simulink model "gabelstapler_Simulink_25a"  (R2025a)
settings: Solver=VariableStepAuto  StartTime=0.0  StopTime=100  RelTol=1e-3
undefined symbols (not defined in the file): d, d_gtr, i_Getriebe, k, K_D, k_e, k_I, k_Motor, k_P, L_Motor, m_fz, m_g, m_gabel, R_Motor, r_R, theta_red, Wirkungsgad_Getriebe
settings Model: Creator=Manuel  LastModifiedBy=gerke

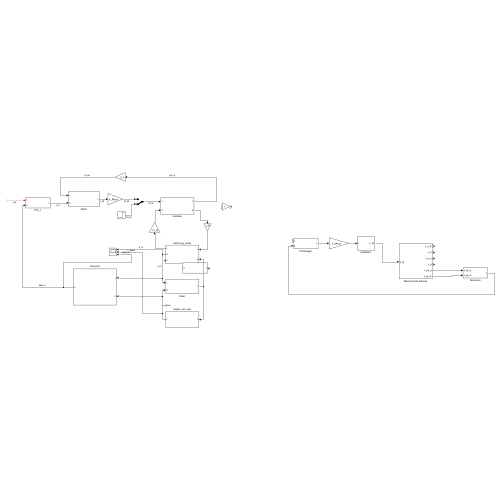
[thumbnail: Simulink's stored preview of the top-level diagram]
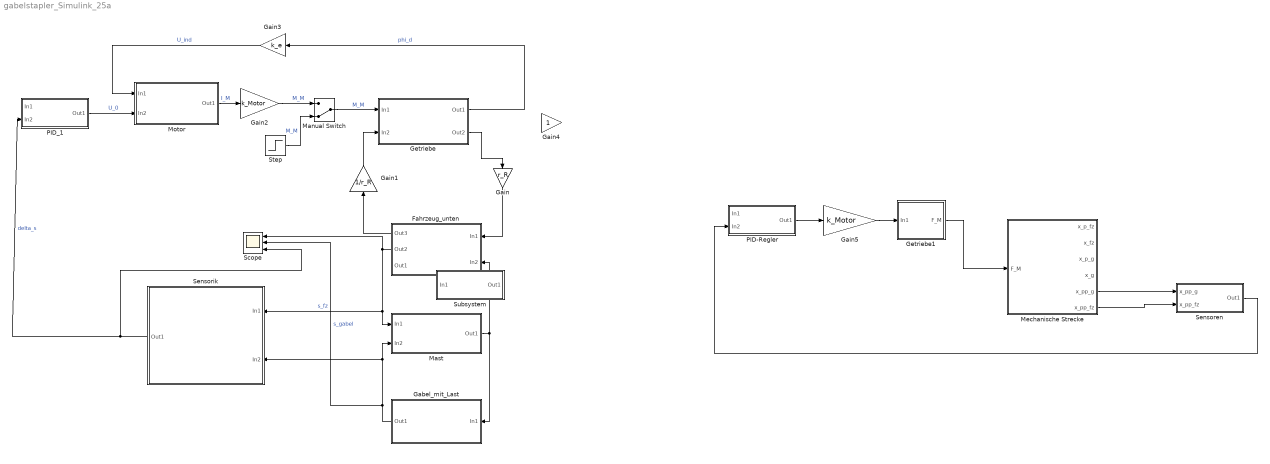
== system gabelstapler_Simulink_25a ==
  Fahrzeug_unten : Subsystem
  Gabel_mit_Last : Subsystem
  Gain : Gain  Gain=r_R
  Gain1 : Gain  Gain=1/r_R
  Gain2 : Gain  Gain=k_Motor
  Gain3 : Gain  Gain=k_e
  Gain4 : Gain
  Gain5 : Gain  Gain=k_Motor
  Getriebe : Subsystem
  Getriebe1 : Subsystem
  Manual Switch : ManualSwitch  CurrentSetting=0
  Mast : Subsystem
  Mechanische Strecke : Subsystem
  Motor : Subsystem
  PID-Regler : Subsystem
  PID_1 : Subsystem
  Scope : Scope  NumInputPorts=3
      settings: ActiveDisplayYMinimum=-3.9889329420410252E+301  ActiveDisplayYMaximum=4.4321477133789155E+300
  Sensoren : Subsystem
  Sensorik : Subsystem
  Step : Step  SampleTime=0
  Subsystem : Subsystem
  wires:
  Gain3/1 -> Motor/1(In1)  "U_ind"
  PID_1/1(Out1) -> Motor/2(In2)  "U_0"
  Motor/1(Out1) -> Gain2/1  "I_M"
  Manual Switch/1 -> Getriebe/1(In1)  "M_M"
  Getriebe/1(Out1) -> Gain3/1  "phi_d"
  Getriebe/2(Out2) -> Gain/1
  Gain/1 -> Fahrzeug_unten/1(In1)
  Fahrzeug_unten/1(Out3) -> Gain1/1
  Gain1/1 -> Getriebe/2(In2)
  Fahrzeug_unten/2(Out2) -> Sensorik/1(In1), Mast/1(In1), Scope/1  "s_fz"
  Gabel_mit_Last/1(Out1) -> Scope/2, Mast/2(In2), Sensorik/2(In2)  "s_gabel"
  Mast/1(Out1) -> Gabel_mit_Last/1(In1), Fahrzeug_unten/2(In2)
  Sensorik/1(Out1) -> Scope/3, PID_1/2(In2)  "delta_s"
  ? -> PID_1/1(In1)  "soll"
  Step/1 -> Manual Switch/2  "M_M"
  Gain2/1 -> Manual Switch/1  "M_M"
  PID-Regler/1(Out1) -> Gain5/1
  Gain5/1 -> Getriebe1/1(In1)
  Getriebe1/1(F_M) -> Mechanische Strecke/1(F_M)
  Mechanische Strecke/5(x_pp_g) -> Sensoren/1(x_pp_g)
  Mechanische Strecke/6(x_pp_fz) -> Sensoren/2(x_pp_fz)
  Sensoren/1(Out1) -> PID-Regler/2(In2)

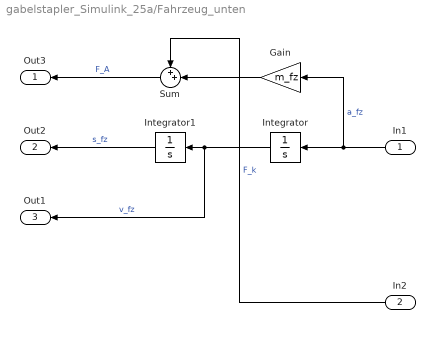
== system gabelstapler_Simulink_25a/Fahrzeug_unten ==
  In1 : Inport
  In2 : Inport  Port=2
  Gain : Gain  Gain=m_fz
  Integrator : Integrator
  Integrator1 : Integrator
  Sum : Sum  Inputs=++|
  Out3 : Outport
  Out2 : Outport  Port=2
  Out1 : Outport  Port=3
  wires:
  Integrator/1 -> Out1/1, Integrator1/1  "v_fz"
  Integrator1/1 -> Out2/1  "s_fz"
  In1/1 -> Integrator/1, Gain/1  "a_fz"
  Sum/1 -> Out3/1  "F_A"
  In2/1 -> Sum/1  "F_k"
  Gain/1 -> Sum/2

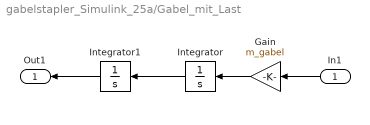
== system gabelstapler_Simulink_25a/Gabel_mit_Last ==
  In1 : Inport
  Gain : Gain  Gain=m_gabel
  Integrator : Integrator
  Integrator1 : Integrator
  Out1 : Outport
  wires:
  Integrator/1 -> Integrator1/1
  In1/1 -> Gain/1
  Integrator1/1 -> Out1/1
  Gain/1 -> Integrator/1

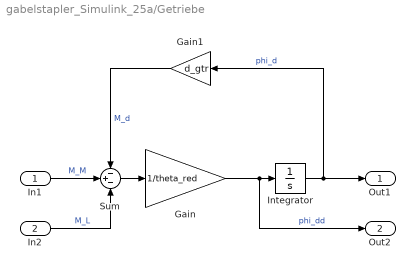
== system gabelstapler_Simulink_25a/Getriebe ==
  In1 : Inport
  In2 : Inport  Port=2
  Gain : Gain  Gain=1/theta_red
  Gain1 : Gain  Gain=d_gtr
  Integrator : Integrator
  Sum : Sum  Inputs=-+-
  Out1 : Outport
  Out2 : Outport  Port=2
  wires:
  Sum/1 -> Gain/1
  Gain/1 -> Integrator/1, Out2/1  "phi_dd"
  Integrator/1 -> Out1/1, Gain1/1  "phi_d"
  Gain1/1 -> Sum/1  "M_d"
  In1/1 -> Sum/2  "M_M"
  In2/1 -> Sum/3  "M_L"

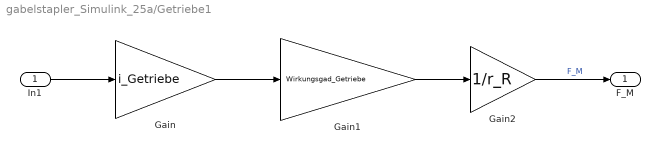
== system gabelstapler_Simulink_25a/Getriebe1 ==
  In1 : Inport
  Gain : Gain  Gain=i_Getriebe
  Gain1 : Gain  Gain=Wirkungsgad_Getriebe
  Gain2 : Gain  Gain=1/r_R
  F_M : Outport
  wires:
  In1/1 -> Gain/1
  Gain/1 -> Gain1/1
  Gain1/1 -> Gain2/1
  Gain2/1 -> F_M/1  "F_M"

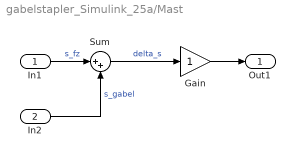
== system gabelstapler_Simulink_25a/Mast ==
  In1 : Inport
  In2 : Inport  Port=2
  Gain : Gain
  Sum : Sum  Inputs=|++
  Out1 : Outport
  wires:
  Sum/1 -> Gain/1  "delta_s"
  In1/1 -> Sum/1  "s_fz"
  Gain/1 -> Out1/1
  In2/1 -> Sum/2  "s_gabel"

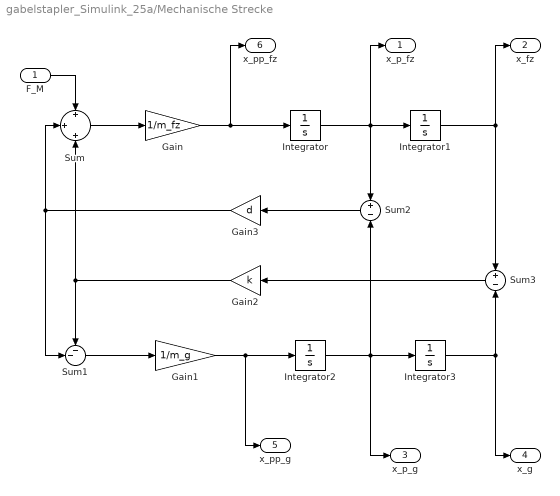
== system gabelstapler_Simulink_25a/Mechanische Strecke ==
  F_M : Inport
  Gain : Gain  Gain=1/m_fz
  Gain1 : Gain  Gain=1/m_g
  Gain2 : Gain  Gain=k
  Gain3 : Gain  Gain=d
  Integrator{,1..3} (4 alike) : Integrator
  Sum : Sum  Inputs=+|+|+
  Sum1 : Sum  Inputs=--|
  Sum2 : Sum  Inputs=+|-
  Sum3 : Sum  Inputs=+|-
  x_p_fz : Outport
  x_fz : Outport  Port=2
  x_p_g : Outport  Port=3
  x_g : Outport  Port=4
  x_pp_g : Outport  Port=5
  x_pp_fz : Outport  Port=6
  wires:
  Sum/1 -> Gain/1
  F_M/1 -> Sum/1
  Integrator/1 -> Sum2/1, Integrator1/1, x_p_fz/1
  Integrator1/1 -> Sum3/1, x_fz/1
  Integrator2/1 -> x_p_g/1, Integrator3/1, Sum2/2
  Integrator3/1 -> x_g/1, Sum3/2
  Sum1/1 -> Gain1/1
  Gain1/1 -> x_pp_g/1, Integrator2/1
  Gain/1 -> x_pp_fz/1, Integrator/1
  Sum3/1 -> Gain2/1
  Sum2/1 -> Gain3/1
  Gain3/1 -> Sum1/2, Sum/2
  Gain2/1 -> Sum1/1, Sum/3

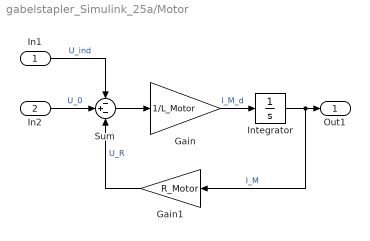
== system gabelstapler_Simulink_25a/Motor ==
  In1 : Inport
  In2 : Inport  Port=2
  Gain : Gain  Gain=1/L_Motor
  Gain1 : Gain  Gain=R_Motor
  Integrator : Integrator
  Sum : Sum  Inputs=-+-
  Out1 : Outport
  wires:
  Gain1/1 -> Sum/3  "U_R"
  Sum/1 -> Gain/1
  In2/1 -> Sum/2  "U_0"
  In1/1 -> Sum/1  "U_ind"
  Integrator/1 -> Gain1/1, Out1/1  "I_M"
  Gain/1 -> Integrator/1  "I_M_d"

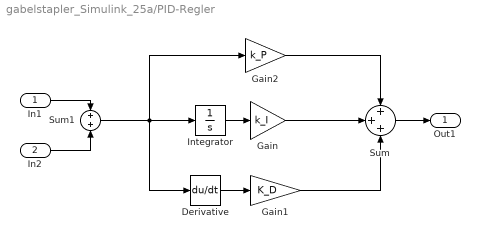
== system gabelstapler_Simulink_25a/PID-Regler ==
  In1 : Inport
  In2 : Inport  Port=2
  Derivative : Derivative
  Gain : Gain  Gain=k_I
  Gain1 : Gain  Gain=K_D
  Gain2 : Gain  Gain=k_P
  Integrator : Integrator
  Sum : Sum  Inputs=+++
  Sum1 : Sum  Inputs=+|+
  Out1 : Outport
  wires:
  Integrator/1 -> Gain/1
  Gain/1 -> Sum/2
  Sum/1 -> Out1/1
  Derivative/1 -> Gain1/1
  Gain1/1 -> Sum/3
  Gain2/1 -> Sum/1
  In2/1 -> Sum1/2
  In1/1 -> Sum1/1
  Sum1/1 -> Integrator/1, Derivative/1, Gain2/1

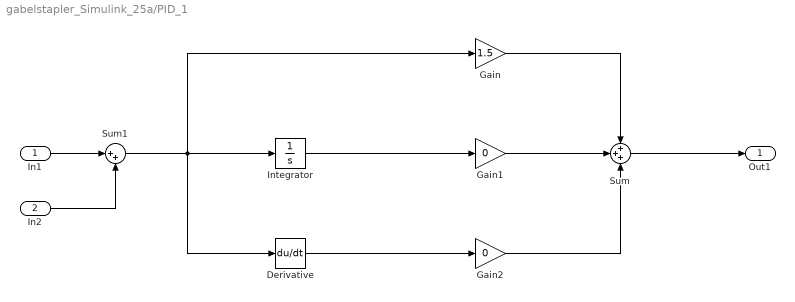
== system gabelstapler_Simulink_25a/PID_1 ==
  In1 : Inport
  In2 : Inport  Port=2
  Derivative : Derivative
  Gain : Gain  Gain=1.5
  Gain1 : Gain  Gain=0
  Gain2 : Gain  Gain=0
  Integrator : Integrator
  Sum : Sum  Inputs=+++
  Sum1 : Sum  Inputs=|++
  Out1 : Outport
  wires:
  Integrator/1 -> Gain1/1
  Derivative/1 -> Gain2/1
  Gain1/1 -> Sum/2
  Gain/1 -> Sum/1
  Gain2/1 -> Sum/3
  Sum/1 -> Out1/1
  In1/1 -> Sum1/1
  Sum1/1 -> Integrator/1, Derivative/1, Gain/1
  In2/1 -> Sum1/2

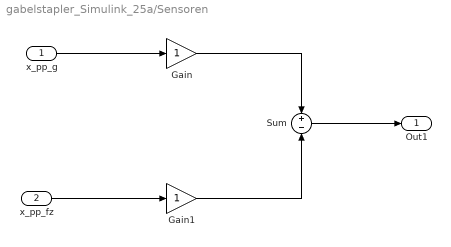
== system gabelstapler_Simulink_25a/Sensoren ==
  x_pp_g : Inport
  x_pp_fz : Inport  Port=2
  Gain : Gain
  Gain1 : Gain
  Sum : Sum  Inputs=+|-
  Out1 : Outport
  wires:
  x_pp_g/1 -> Gain/1
  x_pp_fz/1 -> Gain1/1
  Gain/1 -> Sum/1
  Gain1/1 -> Sum/2
  Sum/1 -> Out1/1

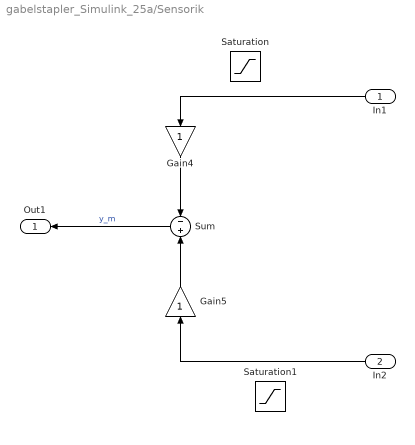
== system gabelstapler_Simulink_25a/Sensorik ==
  In1 : Inport
  In2 : Inport  Port=2
  Gain4 : Gain
  Gain5 : Gain
  Saturation : Saturate
  Saturation1 : Saturate
  Sum : Sum  Inputs=-|+
  Out1 : Outport
  wires:
  In1/1 -> Gain4/1
  In2/1 -> Gain5/1
  Sum/1 -> Out1/1  "y_m"
  Gain5/1 -> Sum/2
  Gain4/1 -> Sum/1

== system gabelstapler_Simulink_25a/Subsystem ==
  In1 : Inport
  Out1 : Outport
  wires:
  In1/1 -> Out1/1
